simulink model "pendulum_cart"  (R2025a)
settings: Solver=ode5  StartTime=0.0  StopTime=30  FixedStep=h  RelTol=1e-3  AbsTol=1e-6
values from neighbouring files (symbols this model uses):
  K = dlqr(Ad,Bd,Q_lqr,R_lqr)    [main.m]
  Ki = K_aug(5)    [main.m]
  Kx = K_aug(1:4)    [main.m]
  Ts = 0.01    [main.m]
  ue = -kd/k1    (= 0.00767069515042)    [main.m]
  xe = [0; pi; 0; 0]    [main.m]
undefined symbols (not defined in the file or in its folder): DiscIntNeverNeededParam, Discrete, Time
libraries: simulink x2, ctrlSharedLib x1
settings Model: SimulationMode=external  ExtModeTrigDuration=12000  ExtModeTrigLevel=0.400000  Creator=jims  LastModifiedBy=kadiraksu
settings SolverCC: AutoScaleAbsTol=off  AlgebraicLoopSolver=TrustRegion
settings DataIOCC: ExternalInput=[]  InitialState=[]  MaxDataPoints=5000  SaveFormat=Array  SignalLoggingSaveFormat=ModelDataLogs  SaveOutput=off  SaveTime=off  ReturnWorkspaceOutputs=off  SignalLoggingName=sigsOut
settings OptimizationCC: BooleanDataType=off  ExpressionDepthLimit=2147483647.0  InitFltsAndDblsToZero=on  LifeSpan=inf
settings DebuggingCC: SaveWithParameterizedLinksMsg=none  UnderspecifiedInitializationDetection=Classic  MergeDetectMultiDrivingBlocksExec=none  SignalResolutionControl=TryResolveAllWithWarning  MultiTaskDSMMsg=warning  MultiTaskCondExecSysMsg=none  IntegerOverflowMsg=none  FcnCallInpInsideContextMsg=warning  UnconnectedInputMsg=warning  UnconnectedOutputMsg=warning  UnconnectedLineMsg=warning  StateNameClashWarn=warning  SFUnexpectedBacktrackingDiag=warning  SFNoUnconditionalDefaultTransitionDiag=warning  SFExecutionAtInitializationDiag=none  IntegerSaturationMsg=none  ArithmeticOperatorsInVariantConditions=warning
settings HardwareCC: ProdBitPerPointer=32.0  ProdBitPerSizeT=32.0  ProdBitPerPtrDiffT=32.0  ProdLargestAtomicFloat=None  ProdIntDivRoundTo=Undefined  ProdEndianess=Unspecified  ProdWordSize=32.0  ProdHWDeviceType=32-bit Generic  TargetBitPerLong=64.0  TargetBitPerPointer=64.0  TargetBitPerSizeT=64.0  TargetBitPerPtrDiffT=64.0  TargetLongLongMode=on  TargetIntDivRoundTo=Zero  TargetEndianess=LittleEndian  TargetWordSize=64.0  TargetHWDeviceType=MATLAB Host  ProdEqTarget=off
settings ModelReferenceCC: EnableRefExpFcnMdlSchedulingChecks=on  PropagateSignalLabelsOutOfModel=off
settings SFSimCC: SimUseLocalCustomCode=off  CustomCodeUndefinedFunction=UseInterfaceOnly
settings RTWCC: SystemTargetFile=rtcon_pendulum_usb2.tlc  TemplateMakefile=rtcon_pendulum_vc_usb2_x64.tmf  RTWUseLocalCustomCode=off  GPUComputeCapability=3.5  DLArmComputeVersion=19.05
settings CodeAppCC: StateflowObjectComments=on
settings STFCustomTargetCC: SystemTargetFile=rtcon_pendulum_usb2.tlc  MultiwordLength=2048.0  DynamicStringBufferSize=256.0  ModelReferenceCompliant=off  CombineOutputUpdateFcns=on  MatFileLogging=on  CPPClassGenCompliant=on  GRTInterface=off  Use_HIGH_PRIORITY=off  StartupMessage=on  Use_REALTIME_PRIORITY=off  LinkRTDACPCI=off  LinkRTDACUSB=off
settings GRTTargetCC: ExtMode=on  ExtModeMexFile=rtcon_ext_comm  TargetLangStandard=C89/C90 (ANSI)  ModelReferenceCompliant=off  ParMdlRefBuildCompliant=off  CompOptLevelCompliant=off  ConcurrentExecutionCompliant=off  UseToolchainInfoCompliant=off
settings ConfigComp: CovMetricSettings=dw  CovSaveCumulativeToWorkspaceVar=on  CovSaveSingleToWorkspaceVar=on  CovExternalEMLEnable=off  CovSFcnEnable=off
settings SimscapeCC: SimscapeLogDecimation=1  SimscapeLogDataHistory=5000

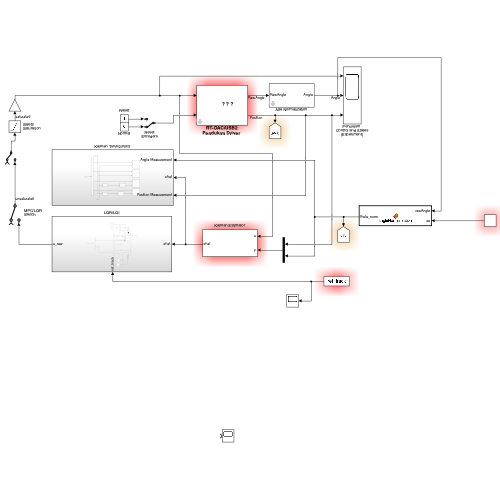
[thumbnail: Simulink's stored preview of the top-level diagram]
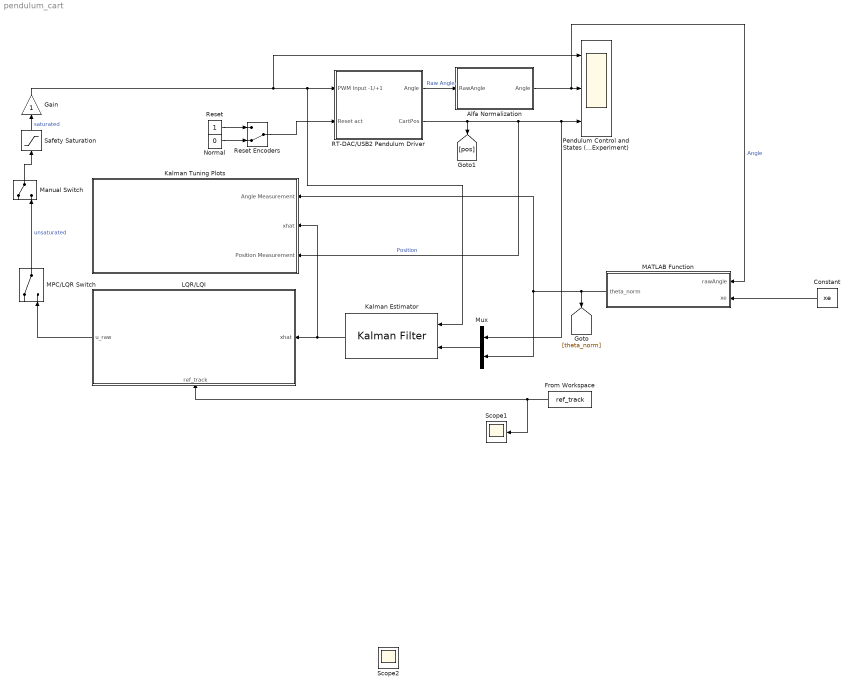
== system pendulum_cart ==
  Alfa Normalization : Subsystem  mask(Choose mode:){pos=Crane Controller}
      mask prompts: pos "Choose mode:"
      mask TypeOptions pos: Inverted Pendulum | Crane Controller
  Constant : Constant  Value=xe  VectorParams1D=off
  From Workspace : FromWorkspace  VariableName=ref_track  SampleTime=Ts
  Gain : Gain
  Kalman Estimator : ctrlSharedLib/Kalman Filter  TimeDomain=Discrete-Time  UseCurrentEstimator=on  ModelSource=LTI State-Space Variable  ModelSourceVariable=sys_d  A=0.95  B=1  C=1  D=0  NumberOfStates=1  NumberOfInputs=1  NumberOfOutputs=1  InitialEstimateSource=Dialog  X0=[0;0;0;0]  P0=10  UseK=off  UseGH=off  NumberOfProcessNoiseInputs=1  G=1  TimeInvariantG=on  H=0  TimeInvariantH=on  Q=[1e-4 1e-2 1.5e2 1.5e2]  TimeInvariantQ=on  R=[1e-6 1e-6]  TimeInvariantR=on  N=0  TimeInvariantN=on  AddInputPort=on  AddEnablePort=off  OutputEstimatedY=off  OutputP=off  Ts=-1
  Kalman Tuning Plots : Subsystem
  LQR/LQI : Subsystem
      settings: PortSchema="{\"entries\":[{\"content\":{\"sides\":[{\"content\":{\"connectorIds\":[\"In1\"]},\"type\":\"ConnectorPlacement.EquallySpacedRectSide\",\"uuid\":\"f28cbfc9-9377-481f-8d61-749de9d5be12\"},{\"content\":{\"connectorIds\":[\"Out1\"],\"side\":\"RIGHT\"},\"type\":\"ConnectorPlacement.EquallySpacedRectSide\",\"uuid\":\"47c89a5d-f617-47ee-b263-77314ba9e5ac\"},{\"content\":{\"connectorIds\":[],\"side\":\"TOP\"},\"type\":\"ConnectorPlacement.EquallySpacedRectSide\",\"uuid\":\"1b28040f-5ded-44df-bd0f-cb2f934e4581\"},{\"content\":{\"connectorIds\":[\"In2\"],\"side\":\"BOTTOM\"},\"type\":\"ConnectorPlacement.EquallySpacedRectSide\",\"uuid\":\"22af4583-4f61-4c59-b79e-ad88b9d70708\"}]},\"type\":\"ConnectorPlacement.EquallySpacedConnector\",\"uuid\":\"31b47320-3909-4a62-82ab-cecd54d18dde\"}],\"packageUris\":[\"http://schema.mathworks.com/mf0/Connector/R2020b\"],\"version\":\"1.0\"}"
  MATLAB Function : MATLAB Function  TreatAsAtomicUnit=on
  MPC/LQR Switch : ManualSwitch
  Manual Switch : ManualSwitch
  Mux : Mux  Inputs=2
  Normal : Constant  Value=0
  Pendulum Control and States (Experiment) : Scope  NumInputPorts=3
      settings: TimeSpan=30  ActiveDisplayYMinimum=-0.9375  ActiveDisplayYMaximum=0.9375  DataLoggingMaxPoints=50000  DataLoggingVariableName=inverted_pendulum_scope_data
  "RT-DAC/USB2 Pendulum Driver " : Subsystem  mask{BoardID=-1, T0=Ts}
      mask prompts: BoardID "Board ID:"; T0 "Sample time:"
      mask help:
      | Serial number of the RT-DAC/USB2 board (BoardID). If only the single board is connected the Board ID should be -1.
      | Sanple time of the real-time executable.
      mask Display: image(imread('pendulum1.jpeg'))
  Reset : Constant
  Reset Encoders : ManualSwitch  CurrentSetting=0
  Safety Saturation : Saturate  UpperLimit=0.75  LowerLimit=-0.75
  Scope1 : Scope
      settings: ActiveDisplayYMinimum=-0.875  ActiveDisplayYMaximum=0.875  DataLoggingVariableName=ScopeData5
  Scope2 : Scope
      settings: ActiveDisplayYMinimum=-15.78261  ActiveDisplayYMaximum=2.23939  DataLoggingVariableName=ScopeData2
  wires:
  "RT-DAC/USB2 Pendulum Driver "/1(Angle) -> Alfa Normalization/1(RawAngle)  "Raw Angle"
  Alfa Normalization/1(Angle) -> MATLAB Function/1(rawAngle), Pendulum Control and States (Experiment)/2  "Angle"
  Reset/1 -> Reset Encoders/1
  Normal/1 -> Reset Encoders/2
  Reset Encoders/1 -> "RT-DAC/USB2 Pendulum Driver "/2(Reset act)
  Gain/1 -> Pendulum Control and States (Experiment)/1, "RT-DAC/USB2 Pendulum Driver "/1(PWM Input -1/+1), Kalman Estimator/1
  Constant/1 -> MATLAB Function/2(xe)
  MATLAB Function/1(theta_norm) -> Mux/2, Kalman Tuning Plots/1(Angle Measurement), [theta_norm]
  "RT-DAC/USB2 Pendulum Driver "/2(CartPos) -> [pos], Pendulum Control and States (Experiment)/3, Mux/1, Kalman Tuning Plots/3(Position Measurement)  "Position"
  Safety Saturation/1 -> Gain/1  "saturated"
  Kalman Estimator/1 -> LQR/LQI/1(xhat), Kalman Tuning Plots/2(xhat)
  Mux/1 -> Kalman Estimator/2
  MPC/LQR Switch/1 -> Manual Switch/2  "unsaturated"
  From Workspace/1 -> Scope1/1, LQR/LQI/2(ref_track)
  LQR/LQI/1(u_raw) -> MPC/LQR Switch/2
  Manual Switch/1 -> Safety Saturation/1

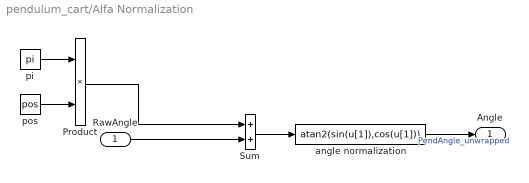
== system pendulum_cart/Alfa Normalization ==
  RawAngle : Inport
  Product : Product  InputSameDT=on  SaturateOnIntegerOverflow=on  OutDataTypeStr=Inherit: Same as first input
  Sum : Sum  InputSameDT=on  SaturateOnIntegerOverflow=on  OutDataTypeStr=Inherit: Same as first input
  angle normalization : Fcn  Expr=atan2(sin(u[1]),cos(u[1]))
  pi : Constant  Value=pi
  pos : Constant  Value=pos
  Angle : Outport  InitialOutput=0  VectorParamsAs1DForOutWhenUnconnected=off
  wires:
  angle normalization/1 -> Angle/1  "PendAngle_unwrapped"
  Sum/1 -> angle normalization/1
  RawAngle/1 -> Sum/2
  pi/1 -> Product/1
  pos/1 -> Product/2
  Product/1 -> Sum/1

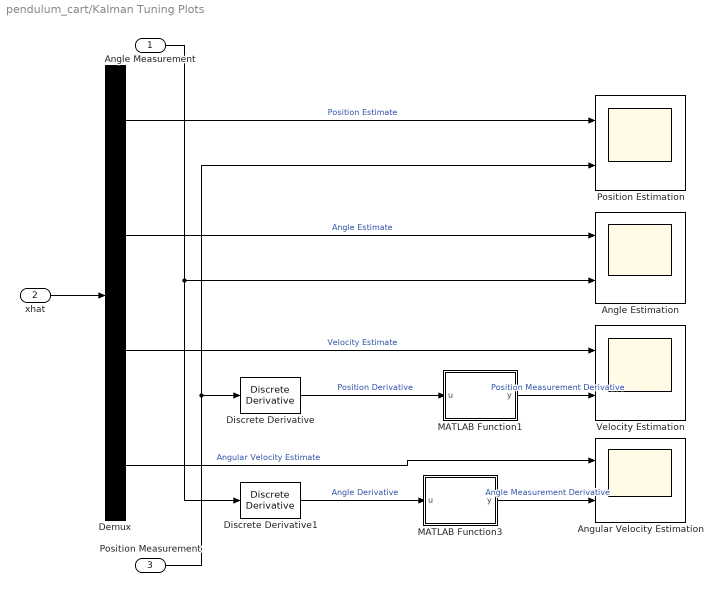
== system pendulum_cart/Kalman Tuning Plots ==
  Angle Measurement : Inport
  xhat : Inport  Port=2
  Position Measurement : Inport  Port=3
  Angle Estimation : Scope  NumInputPorts=2
      settings: ActiveDisplayYMinimum=-2.23616  ActiveDisplayYMaximum=2.08583  DataLoggingVariableName=ScopeData2
  Angular Velocity Estimation : Scope  NumInputPorts=2
      settings: ActiveDisplayYMinimum=-10.52608  ActiveDisplayYMaximum=10.62124  DataLoggingVariableName=ScopeData2
  Demux : Demux
  Discrete Derivative : simulink/Discrete/Discrete Derivative  gainval=1.0  ICPrevScaledInput=0.0  OutMin=[]  OutMax=[]  OutDataType=fixdt(1, 16)  OutScaling=2^-10  DoSatur=off
  Discrete Derivative1 : simulink/Discrete/Discrete Derivative  gainval=1.0  ICPrevScaledInput=0.0  OutMin=[]  OutMax=[]  OutDataType=fixdt(1, 16)  OutScaling=2^-10  DoSatur=off
  MATLAB Function1 : MATLAB Function  TreatAsAtomicUnit=on
  MATLAB Function3 : MATLAB Function  TreatAsAtomicUnit=on
  Position Estimation : Scope  NumInputPorts=2
      settings: ActiveDisplayYMinimum=-0.90235  ActiveDisplayYMaximum=0.84507  DataLoggingVariableName=ScopeData3
  Velocity Estimation : Scope  NumInputPorts=2
      settings: ActiveDisplayYMinimum=-1.50086  ActiveDisplayYMaximum=1.51171
  wires:
  Demux/3 -> Velocity Estimation/1  "Velocity Estimate"
  Angle Measurement/1 -> Angle Estimation/2, Discrete Derivative1/1
  Demux/4 -> Angular Velocity Estimation/1  "Angular Velocity Estimate"
  Position Measurement/1 -> Discrete Derivative/1, Position Estimation/2
  MATLAB Function1/1(y) -> Velocity Estimation/2  "Position Measurement Derivative"
  Discrete Derivative/1 -> MATLAB Function1/1(u)  "Position Derivative"
  MATLAB Function3/1(y) -> Angular Velocity Estimation/2  "Angle Measurement Derivative"
  Discrete Derivative1/1 -> MATLAB Function3/1(u)  "Angle Derivative"
  Demux/2 -> Angle Estimation/1  "Angle Estimate"
  Demux/1 -> Position Estimation/1  "Position Estimate"
  xhat/1 -> Demux/1

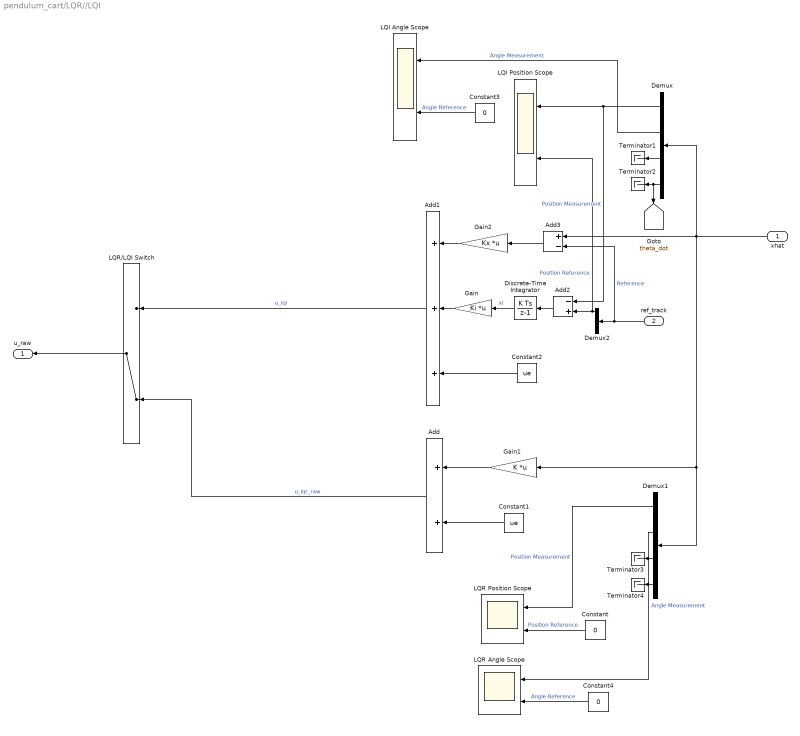
== system pendulum_cart/LQR//LQI ==
  xhat : Inport
  ref_track : Inport  Port=2
  Add : Sum
  Add1 : Sum  Inputs=+++
  Add2 : Sum  Inputs=-+
  Add3 : Sum  Inputs=+-
  Constant : Constant  Value=0  VectorParams1D=off
  Constant1 : Constant  Value=ue  VectorParams1D=off
  Constant2 : Constant  Value=ue  VectorParams1D=off
  Constant3 : Constant  Value=0  VectorParams1D=off
  Constant4 : Constant  Value=0  VectorParams1D=off
  Demux : Demux
  Demux1 : Demux
  Demux2 : Demux
  Discrete-Time Integrator : DiscreteIntegrator  SampleTime=Ts  ICPrevOutput=DiscIntNeverNeededParam  ICPrevScaledInput=DiscIntNeverNeededParam
  Gain : Gain  Gain=Ki  Multiplication=Matrix(K*u)
  Gain1 : Gain  Gain=K  Multiplication=Matrix(K*u)
  Gain2 : Gain  Gain=Kx  Multiplication=Matrix(K*u)
  LQI Angle Scope : Scope  NumInputPorts=2
      settings: ActiveDisplayYMinimum=-3.91431  ActiveDisplayYMaximum=3.92225  DataLoggingVariableName=lqrAngleComp
  LQI Position Scope : Scope  NumInputPorts=2
      settings: ActiveDisplayYMinimum=-0.4759  ActiveDisplayYMaximum=0.83065  DataLoggingVariableName=lqrPositionComp
  LQR Angle Scope : Scope  NumInputPorts=2
      settings: ActiveDisplayYMinimum=-0.12847  ActiveDisplayYMaximum=0.09779  DataLoggingVariableName=ScopeData8
  LQR Position Scope : Scope  NumInputPorts=2
      settings: ActiveDisplayYMinimum=-0.162  ActiveDisplayYMaximum=0.19936  DataLoggingVariableName=ScopeData7
  LQR/LQI Switch : ManualSwitch  CurrentSetting=0
  Terminator{1..4} (4 alike) : Terminator
  u_raw : Outport
  tag scope: theta_dot=global
  wires:
  LQR/LQI Switch/1 -> u_raw/1
  Gain2/1 -> Add1/1
  Add1/1 -> LQR/LQI Switch/1  "u_lqi"
  Add/1 -> LQR/LQI Switch/2  "u_lqr_raw"
  Gain1/1 -> Add/1
  Constant1/1 -> Add/2
  Gain/1 -> Add1/2
  Add2/1 -> Discrete-Time Integrator/1
  Discrete-Time Integrator/1 -> Gain/1  "xi"
  Constant2/1 -> Add1/3
  Demux2/1 -> Add2/2, LQI Position Scope/2  "Position Reference"
  ref_track/1 -> Add3/2, Demux2/1  "Reference"
  xhat/1 -> Add3/1, Demux/1, Demux1/1, Gain1/1
  Add3/1 -> Gain2/1
  Demux/1 -> Add2/1, LQI Position Scope/1  "Position Measurement"
  Demux/2 -> LQI Angle Scope/1  "Angle Measurement"
  Demux/4 -> [theta_dot], Terminator2/1
  Demux/3 -> Terminator1/1
  Demux1/1 -> LQR Position Scope/1  "Position Measurement"
  Demux1/2 -> LQR Angle Scope/1  "Angle Measurement"
  Demux1/3 -> Terminator3/1
  Demux1/4 -> Terminator4/1
  Constant/1 -> LQR Position Scope/2  "Position Reference"
  Constant3/1 -> LQI Angle Scope/2  "Angle Reference"
  Constant4/1 -> LQR Angle Scope/2  "Angle Reference"

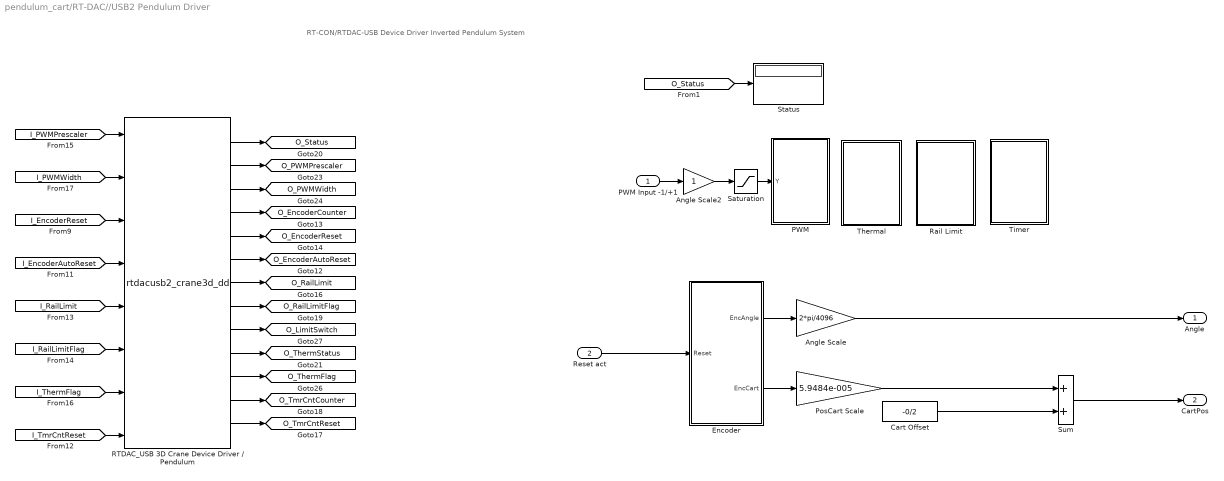
== system pendulum_cart/RT-DAC//USB2 Pendulum Driver  ==
  note: RT-CON/RTDAC-USB Device Driver
      | Inverted Pendulum System
  PWM Input -1/+1 : Inport
  Reset act : Inport  Port=2
  Angle Scale : Gain  Gain=2*pi/4096  OutDataTypeStr=Inherit: Same as input  ParamDataTypeStr=Inherit: Same as input
  Angle Scale2 : Gain  OutDataTypeStr=Inherit: Same as input  ParamDataTypeStr=Inherit: Same as input
  Cart Offset : Constant  Value=-0/2
  Encoder : Subsystem
  PWM : Subsystem
      mask Display: disp('PWM')
  PosCart Scale : Gain  Gain=5.9484e-005  OutDataTypeStr=Inherit: Same as input  ParamDataTypeStr=Inherit: Same as input
  RTDAC_USB 3D Crane Device Driver / Pendulum : S-Function  FunctionName=rtdacusb2_crane3d_dd  Parameters=-1, 0.01  SFunctionDeploymentMode=off  EnableBusSupport=off
  Rail Limit : Subsystem
      mask Display: disp('Rail\nLimit')
  Saturation : Saturate  UpperLimit=1  LowerLimit=-1
  Status : Display
      settings: Format=hex (Stored Integer)
  Sum : Sum  InputSameDT=on  SaturateOnIntegerOverflow=on  OutDataTypeStr=Inherit: Same as first input
  Thermal : Subsystem
      mask Display: disp('Thermal')
  Timer : Subsystem
      mask Display: disp('Timer')
  Angle : Outport  VectorParamsAs1DForOutWhenUnconnected=off
  CartPos : Outport  Port=2  VectorParamsAs1DForOutWhenUnconnected=off
  tag scope: O_EncoderAutoReset=global, O_EncoderCounter=global, O_EncoderReset=global, O_LimitSwitch=global, O_PWMPrescaler=global, O_PWMWidth=global, O_RailLimit=global, O_RailLimitFlag=global, O_Status=global, O_ThermFlag=global, O_ThermStatus=global, O_TmrCntCounter=global, O_TmrCntReset=global
  wires:
  RTDAC_USB 3D Crane Device Driver / Pendulum/4 -> [O_EncoderCounter]
  [I_EncoderAutoReset] -> RTDAC_USB 3D Crane Device Driver / Pendulum/4
  RTDAC_USB 3D Crane Device Driver / Pendulum/7 -> [O_RailLimit]
  [I_RailLimit] -> RTDAC_USB 3D Crane Device Driver / Pendulum/5
  RTDAC_USB 3D Crane Device Driver / Pendulum/6 -> [O_EncoderAutoReset]
  [I_RailLimitFlag] -> RTDAC_USB 3D Crane Device Driver / Pendulum/6
  RTDAC_USB 3D Crane Device Driver / Pendulum/10 -> [O_ThermStatus]
  RTDAC_USB 3D Crane Device Driver / Pendulum/5 -> [O_EncoderReset]
  RTDAC_USB 3D Crane Device Driver / Pendulum/9 -> [O_LimitSwitch]
  [I_EncoderReset] -> RTDAC_USB 3D Crane Device Driver / Pendulum/3
  RTDAC_USB 3D Crane Device Driver / Pendulum/8 -> [O_RailLimitFlag]
  [I_TmrCntReset] -> RTDAC_USB 3D Crane Device Driver / Pendulum/8
  RTDAC_USB 3D Crane Device Driver / Pendulum/3 -> [O_PWMWidth]
  RTDAC_USB 3D Crane Device Driver / Pendulum/13 -> [O_TmrCntReset]
  RTDAC_USB 3D Crane Device Driver / Pendulum/11 -> [O_ThermFlag]
  [I_PWMWidth] -> RTDAC_USB 3D Crane Device Driver / Pendulum/2
  [I_ThermFlag] -> RTDAC_USB 3D Crane Device Driver / Pendulum/7
  [I_PWMPrescaler] -> RTDAC_USB 3D Crane Device Driver / Pendulum/1
  RTDAC_USB 3D Crane Device Driver / Pendulum/1 -> [O_Status]
  RTDAC_USB 3D Crane Device Driver / Pendulum/2 -> [O_PWMPrescaler]
  RTDAC_USB 3D Crane Device Driver / Pendulum/12 -> [O_TmrCntCounter]
  [O_Status] -> Status/1
  PWM Input -1/+1/1 -> Angle Scale2/1
  Reset act/1 -> Encoder/1(Reset)
  Cart Offset/1 -> Sum/2
  Sum/1 -> CartPos/1
  PosCart Scale/1 -> Sum/1
  Saturation/1 -> PWM/1(Y)
  Encoder/2(EncCart) -> PosCart Scale/1
  Encoder/1(EncAngle) -> Angle Scale/1
  Angle Scale2/1 -> Saturation/1
  Angle Scale/1 -> Angle/1

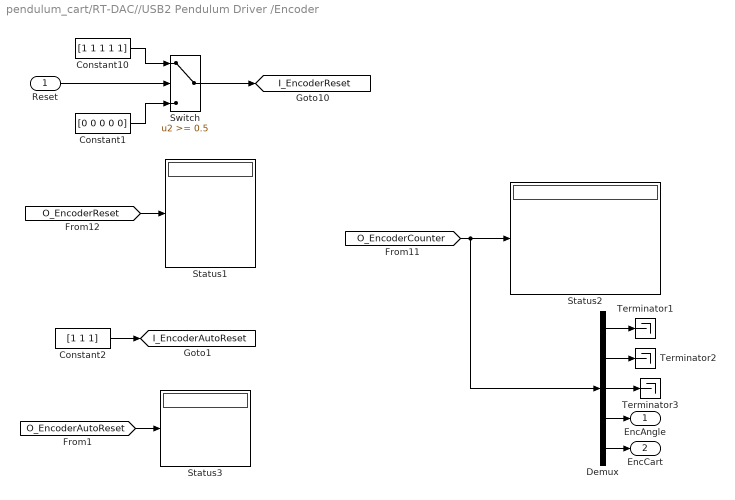
== system pendulum_cart/RT-DAC//USB2 Pendulum Driver /Encoder ==
  Reset : Inport
  Constant1 : Constant  Value=[0 0 0 0 0]
  Constant10 : Constant  Value=[1 1 1 1 1]
  Constant2 : Constant  Value=[1 1 1]
  Demux : Demux  Outputs=5
  Status1 : Display
  Status2 : Display
  Status3 : Display
  Switch : Switch  Threshold=0.5  SaturateOnIntegerOverflow=off
  Terminator1 : Terminator
  Terminator2 : Terminator
  Terminator3 : Terminator
  EncAngle : Outport  VectorParamsAs1DForOutWhenUnconnected=off
  EncCart : Outport  Port=2  VectorParamsAs1DForOutWhenUnconnected=off
  tag scope: I_EncoderAutoReset=global, I_EncoderReset=global
  wires:
  [O_EncoderAutoReset] -> Status3/1
  Constant2/1 -> [I_EncoderAutoReset]
  Demux/5 -> EncCart/1
  Demux/4 -> EncAngle/1
  Constant1/1 -> Switch/3
  Constant10/1 -> Switch/1
  Switch/1 -> [I_EncoderReset]
  Reset/1 -> Switch/2
  Demux/3 -> Terminator3/1
  Demux/2 -> Terminator2/1
  Demux/1 -> Terminator1/1
  [O_EncoderCounter] -> Status2/1, Demux/1
  [O_EncoderReset] -> Status1/1

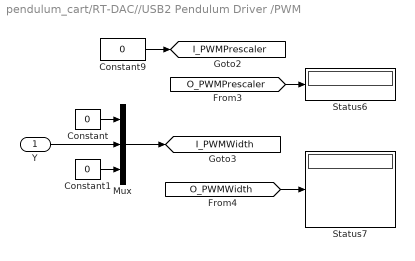
== system pendulum_cart/RT-DAC//USB2 Pendulum Driver /PWM ==
  Y : Inport
  Constant : Constant  Value=0
  Constant1 : Constant  Value=0
  Constant9 : Constant  Value=0
  Mux : Mux  Inputs=3
  Status6 : Display
  Status7 : Display
  tag scope: I_PWMPrescaler=global, I_PWMWidth=global
  wires:
  Constant1/1 -> Mux/3
  Mux/1 -> [I_PWMWidth]
  Y/1 -> Mux/2
  Constant/1 -> Mux/1
  Constant9/1 -> [I_PWMPrescaler]
  [O_PWMPrescaler] -> Status6/1
  [O_PWMWidth] -> Status7/1

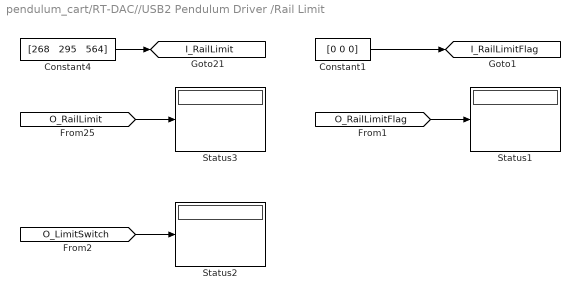
== system pendulum_cart/RT-DAC//USB2 Pendulum Driver /Rail Limit ==
  Constant1 : Constant  Value=[0 0 0]
  Constant4 : Constant  Value="[268   295   564]"
  Status1 : Display
  Status2 : Display
  Status3 : Display
  tag scope: I_RailLimit=global, I_RailLimitFlag=global
  wires:
  [O_LimitSwitch] -> Status2/1
  Constant1/1 -> [I_RailLimitFlag]
  [O_RailLimitFlag] -> Status1/1
  Constant4/1 -> [I_RailLimit]
  [O_RailLimit] -> Status3/1

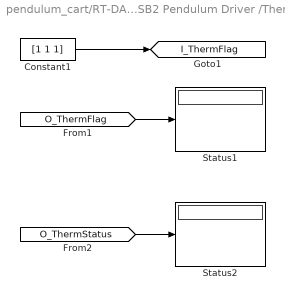
== system pendulum_cart/RT-DAC//USB2 Pendulum Driver /Thermal ==
  Constant1 : Constant  Value=[1 1 1]
  Status1 : Display
  Status2 : Display
  tag scope: I_ThermFlag=global
  wires:
  [O_ThermFlag] -> Status1/1
  Constant1/1 -> [I_ThermFlag]
  [O_ThermStatus] -> Status2/1

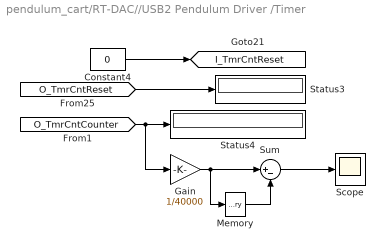
== system pendulum_cart/RT-DAC//USB2 Pendulum Driver /Timer ==
  Constant4 : Constant  Value=0
  Gain : Gain  Gain=1/40000  SaturateOnIntegerOverflow=on  OutDataTypeStr=Inherit: Same as input  ParamDataTypeStr=Inherit: Same as input
  Memory : Memory
  Scope : Scope
      settings: TimeSpan=10  ActiveDisplayYMinimum=0  ActiveDisplayYMaximum=30
  Status3 : Display
  Status4 : Display
  Sum : Sum  Inputs=|+-  InputSameDT=on  SaturateOnIntegerOverflow=on  OutDataTypeStr=Inherit: Same as first input
  tag scope: I_TmrCntReset=global
  wires:
  Sum/1 -> Scope/1
  Memory/1 -> Sum/2
  Gain/1 -> Memory/1, Sum/1
  [O_TmrCntCounter] -> Gain/1, Status4/1
  [O_TmrCntReset] -> Status3/1
  Constant4/1 -> [I_TmrCntReset]

== matlab function pendulum_cart/MATLAB Function ==
  data: rawAngle input; theta_norm output; xe input
function theta_norm = angleNormalization(rawAngle, xe)

% xe(2) contains the equilibrium angle
% downward model: xe(2) = 0
% upward model:   xe(2) = pi

theta_eq = xe(2);
theta_norm = atan2(sin(rawAngle - theta_eq), cos(rawAngle - theta_eq));

end

== matlab function pendulum_cart/Kalman Tuning Plots/MATLAB Function3 ==
  data: u input; y output
function y = Lowpass_Filter(u)

%#codegen

persistent y_prev

Ts = 0.01;
fc = 20;   % Hz, try 3-8 Hz

alpha = (2*pi*fc*Ts)/(1 + 2*pi*fc*Ts);

if isempty(y_prev)
    y_prev = u;
end

y = y_prev + alpha*(u - y_prev);

y_prev = y;

end

== matlab function pendulum_cart/Kalman Tuning Plots/MATLAB Function1 ==
  data: u input; y output
function y = Lowpass_Filter(u)

%#codegen

persistent y_prev

Ts = 0.01;
fc = 8;   % Hz, try 3-8 Hz

alpha = (2*pi*fc*Ts)/(1 + 2*pi*fc*Ts);

if isempty(y_prev)
    y_prev = u;
end

y = y_prev + alpha*(u - y_prev);

y_prev = y;

end
